simulink model "PNEU_BH"  (R2023a)
settings: Solver=ode14x  StartTime=0.0  StopTime=10  FixedStep=1e-6  RelTol=1e-3
values from neighbouring files (symbols this model uses):
  a = Parameters(4)    [BH_FMIN_WeightedError.m]    (also in BH_FMIN_WeightedError_Main.m = 3.2)
  Aa = 6.91e-4    (= 0.000691)    [PNEU_PARAMETROS.m]
  Ab = 8.94e-4    (= 0.000894)    [PNEU_PARAMETROS.m]
  BH_y = Parameters(2)    [BH_FMIN_WeightedError.m]    (also in BH_FMIN_WeightedError_Main.m = 170)
  Fext = 0    [PNEU_PARAMETROS.m]
  GuA0 = 3.2e3    (= 3200)    [PNEU_PARAMETROS.m]
  GuB0 = 3.2e3    (= 3200)    [PNEU_PARAMETROS.m]
  k1 = Parameters(5)    [BH_FMIN_WeightedError.m]    (also in BH_FMIN_WeightedError_Main.m = 11)
  k2 = Parameters(6)    [BH_FMIN_WeightedError.m]    (also in BH_FMIN_WeightedError_Main.m = 0.9)
  ka = 36    [PNEU_PARAMETROS.m]
  M = 2.7    [PNEU_PARAMETROS.m]
  M0 = Parameters(1)    [BH_FMIN_WeightedError.m]    (also in BH_FMIN_WeightedError_Main.m = 480)
  PA0 = 4.97    [PNEU_PARAMETROS.m]
  PB0 = 5.61    [PNEU_PARAMETROS.m]
  R = 8.314e-5    (= 8.314e-05)    [PNEU_PARAMETROS.m]
  ro = 0.62    [BH_FMIN_WeightedError_Main.m]
  ta = 0.112    [PNEU_PARAMETROS.m]
  TA0 = 293.15    [PNEU_PARAMETROS.m]
  tb = 0.104    [PNEU_PARAMETROS.m]
  TB0 = 293.15    [PNEU_PARAMETROS.m]
  VA0 = 0.2*Aa    (= 0.0001382)    [PNEU_PARAMETROS.m]
  VB0 = 0.2*Ab    (= 0.0001788)    [PNEU_PARAMETROS.m]
  y = sim("PNEU_PID.slx")    [PID_FMIN_WeightedError.m]    (also in PNEU_PARAMETROS.m = 1.4)
settings Model: Creator=AndreiaOliveira  LastModifiedBy=Francisco Stigliano
settings OptimizationCC: ReuseModelBlockBuffer=off

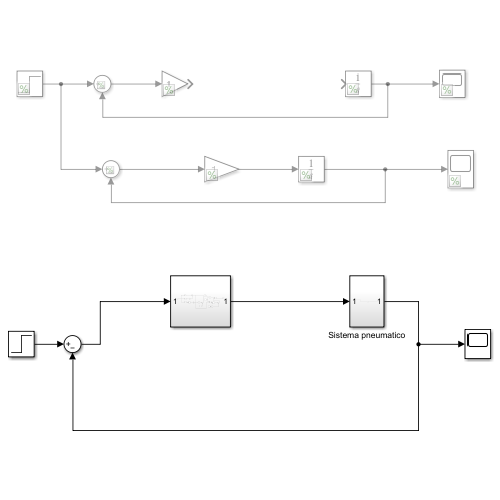
[thumbnail: Simulink's stored preview of the top-level diagram]
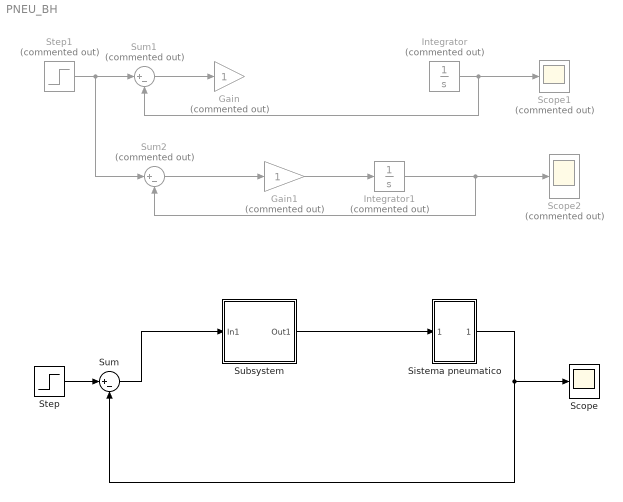
== system PNEU_BH ==
  Gain : Gain  Commented=on
  Gain1 : Gain  Commented=on
  Integrator : Integrator  Commented=on  InitialCondition=1  ZeroCross=off
  Integrator1 : Integrator  Commented=on
  Scope : Scope
  Scope1 : Scope  Commented=on
  Scope2 : Scope  Commented=on
  Sistema pneumatico : Subsystem
  Step : Step  After=0.2  SampleTime=0
  Step1 : Step  Commented=on  SampleTime=0
  Subsystem : Subsystem
  Sum : Sum  Inputs=|+-
  Sum1 : Sum  Commented=on  Inputs=|+-
  Sum2 : Sum  Commented=on  Inputs=|+-
  wires:
  Sistema pneumatico/1(Out1) -> Sum/2, Scope/1
  Step/1 -> Sum/1
  Sum/1 -> Subsystem/1(In1)
  Subsystem/1(Out1) -> Sistema pneumatico/1(In1)
  Integrator1/1 -> Sum2/2, Scope2/1
  Sum1/1 -> Gain/1
  Step1/1 -> Sum2/1, Sum1/1
  Integrator/1 -> Sum1/2, Scope1/1
  Sum2/1 -> Gain1/1
  Gain1/1 -> Integrator1/1

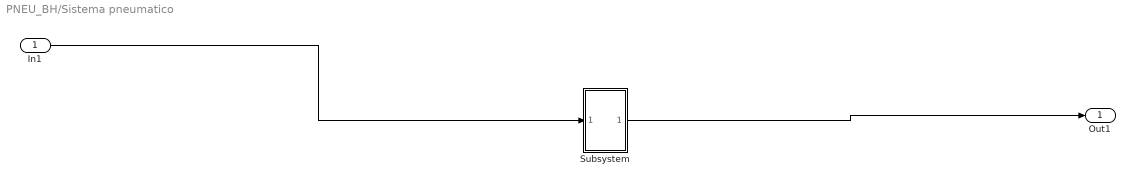
== system PNEU_BH/Sistema pneumatico ==
  In1 : Inport
  Subsystem : Subsystem
  Out1 : Outport
  wires:
  In1/1 -> Subsystem/1(In1)
  Subsystem/1(Out1) -> Out1/1

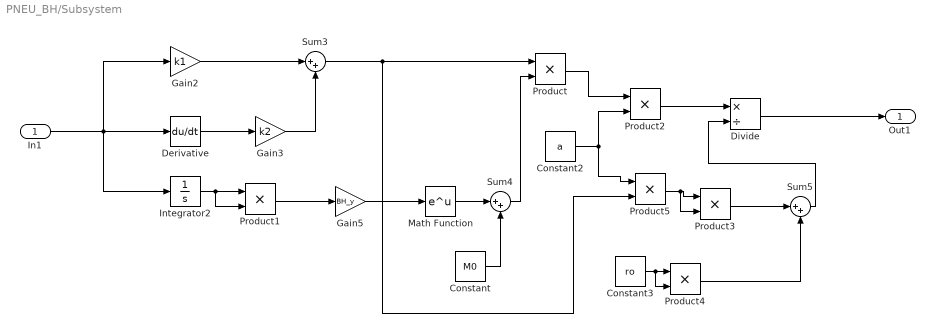
== system PNEU_BH/Subsystem ==
  In1 : Inport
  Constant : Constant  Value=M0
  Constant2 : Constant  Value=a
  Constant3 : Constant  Value=ro
  Derivative : Derivative
  Divide : Product  Inputs=*/
  Gain2 : Gain  Gain=k1
  Gain3 : Gain  Gain=k2
  Gain5 : Gain  Gain=BH_y
  Integrator2 : Integrator
  Math Function : Math
  Product{,1..5} (6 alike) : Product
  Sum3 : Sum  Inputs=|++
  Sum4 : Sum  Inputs=|++
  Sum5 : Sum  Inputs=|++
  Out1 : Outport
  wires:
  Sum5/1 -> Divide/2
  Math Function/1 -> Sum4/1
  Sum3/1 -> Product5/2, Product/1
  Product/1 -> Product2/1
  Divide/1 -> Out1/1
  Constant3/1 -> Product4/2, Product4/1
  Constant2/1 -> Product5/1, Product2/2
  In1/1 -> Integrator2/1, Gain2/1, Derivative/1
  Sum4/1 -> Product/2
  Product5/1 -> Product3/2, Product3/1
  Gain2/1 -> Sum3/1
  Constant/1 -> Sum4/2
  Integrator2/1 -> Product1/2, Product1/1
  Product1/1 -> Gain5/1
  Derivative/1 -> Gain3/1
  Product3/1 -> Sum5/1
  Gain3/1 -> Sum3/2
  Gain5/1 -> Math Function/1
  Product4/1 -> Sum5/2
  Product2/1 -> Divide/1

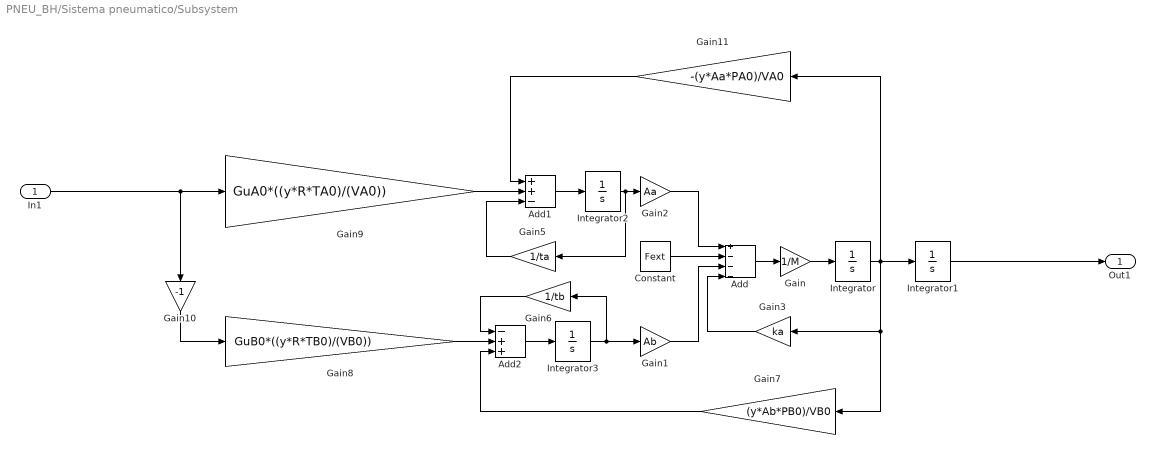
== system PNEU_BH/Sistema pneumatico/Subsystem ==
  In1 : Inport
  Add : Sum  Inputs=+---
  Add1 : Sum  Inputs=++-
  Add2 : Sum  Inputs=-++
  Constant : Constant  Value=Fext
  Gain : Gain  Gain=1/M
  Gain1 : Gain  Gain=Ab
  Gain10 : Gain  Gain=-1
  Gain11 : Gain  Gain=-(y*Aa*PA0)/VA0
  Gain2 : Gain  Gain=Aa
  Gain3 : Gain  Gain=ka
  Gain5 : Gain  Gain=1/ta
  Gain6 : Gain  Gain=1/tb
  Gain7 : Gain  Gain=(y*Ab*PB0)/VB0
  Gain8 : Gain  Gain=GuB0*((y*R*TB0)/(VB0))
  Gain9 : Gain  Gain=GuA0*((y*R*TA0)/(VA0))
  Integrator{,1..3} (4 alike) : Integrator
  Out1 : Outport
  wires:
  Gain7/1 -> Add2/3
  Gain5/1 -> Add1/3
  Constant/1 -> Add/2
  Integrator2/1 -> Gain5/1, Gain2/1
  Integrator1/1 -> Out1/1
  Gain1/1 -> Add/3
  Add1/1 -> Integrator2/1
  Gain10/1 -> Gain8/1
  Gain11/1 -> Add1/1
  In1/1 -> Gain9/1, Gain10/1
  Integrator/1 -> Integrator1/1, Gain11/1, Gain7/1, Gain3/1
  Gain9/1 -> Add1/2
  Add2/1 -> Integrator3/1
  Integrator3/1 -> Gain6/1, Gain1/1
  Gain8/1 -> Add2/2
  Gain6/1 -> Add2/1
  Gain/1 -> Integrator/1
  Gain2/1 -> Add/1
  Gain3/1 -> Add/4
  Add/1 -> Gain/1
